simulink subsystem "hardware"  (R2022a)
settings: Solver=VariableStepAuto  StartTime=0.0  StopTime=10.0  RelTol=1e-3
undefined symbols (not defined in the file or in its folder): HS, IO291
libraries: aru_toolbox x5, eeGeneralControl x4, speedgoatlib_IO691 x3, speedgoatlib_IO291 x1
settings Model: Creator=Mechatronics  LastModifiedBy=Mechatronics

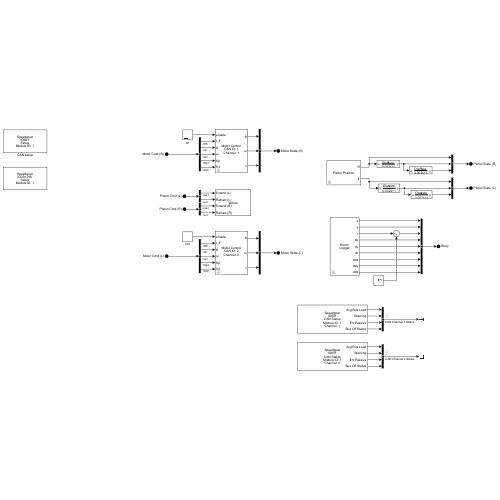
[thumbnail: Simulink's stored preview of the top-level diagram]
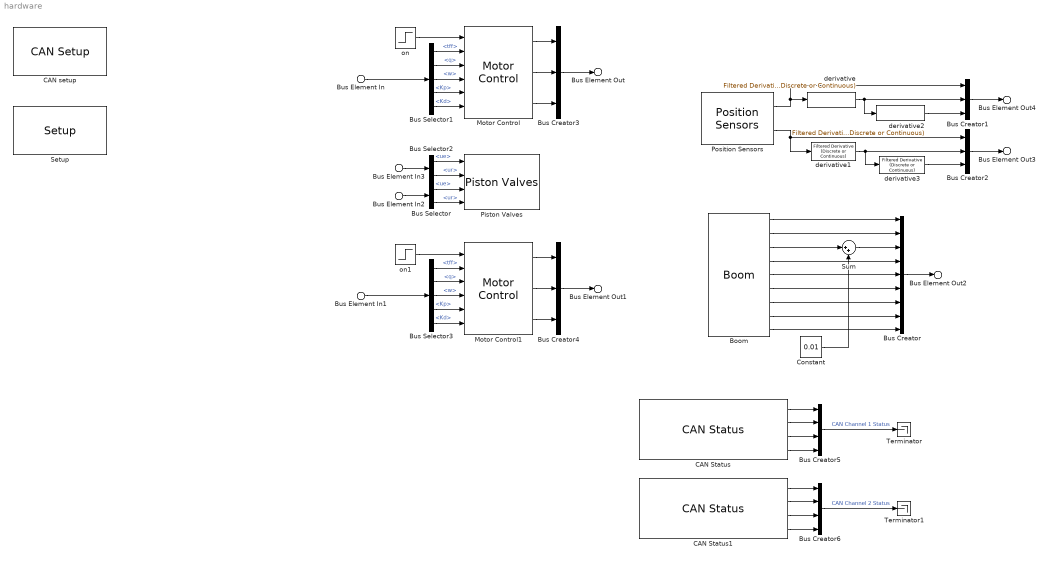
== system hardware ==
  Bus Element In : Inport  PortName=Motor Cmd (R)
  Bus Element In2 : Inport  Port=2  PortName=Piston Cmd (R)
  Bus Element In3 : Inport  Port=3  PortName=Piston Cmd (L)
  Bus Element In1 : Inport  Port=4  PortName=Motor Cmd (L)
  Boom : aru_toolbox/Boom  ts=0.001
      link override Serial Read HW FIFO: pciSlot=-1  board=IO393-50k
      link override Serial Setup: pciSlot=-1  board=IO393-50k
      settings: SourceProductName=ARU Toolbox
  Bus Creator : BusCreator  Inputs=9  OutDataTypeStr=Bus: BodyState  NonVirtualBus=on
      settings: InheritFromInputs=off
  Bus Creator1 : BusCreator  Inputs=3  OutDataTypeStr=Bus: PistonState  NonVirtualBus=on
      settings: InheritFromInputs=off
  Bus Creator2 : BusCreator  Inputs=3  OutDataTypeStr=Bus: PistonState  NonVirtualBus=on
      settings: InheritFromInputs=off
  Bus Creator3 : BusCreator  Inputs=3  OutDataTypeStr=Bus: MotorState  NonVirtualBus=on
      settings: InheritFromInputs=off
  Bus Creator4 : BusCreator  Inputs=3  OutDataTypeStr=Bus: MotorState  NonVirtualBus=on
      settings: InheritFromInputs=off
  Bus Creator5 : BusCreator  Inputs=4  OutDataTypeStr=Bus: CAN  NonVirtualBus=on
      settings: InheritFromInputs=off
  Bus Creator6 : BusCreator  Inputs=4  OutDataTypeStr=Bus: CAN  NonVirtualBus=on
      settings: InheritFromInputs=off
  Bus Selector : BusSelector  OutputSignals=ue,ur
  Bus Selector1 : BusSelector  OutputSignals=tff,q,w,Kp,Kd
  Bus Selector2 : BusSelector  OutputSignals=ue,ur
  Bus Selector3 : BusSelector  OutputSignals=tff,q,w,Kp,Kd
  CAN Status : speedgoatlib_IO691/Legacy/CAN Status  moduleId=1  sampleTime=0.001  channel=1  busRecovery=Auto  arrayOutput=off  controllerCpuLoad=off  controllerLiveCount=off  initModeAct=off  avgBusLoad=on  receiving=off  RxQueueEmpty=off  dataOverrunRcv=off  rxBufferLevel=off  txPending=off  dataOverrunTx=off  txBufferLevel=off  errWarnLimit=on  errPassLimit=on  errBusOff=on  busRecoveryCounter=off  busCouplingErr=off  transceiverErr=off  opMode=off  brp=off  timeSegment1=off  timeSegment2=off  synchronisationJumpWidth=off  dataTSEG1=off  dataTSEG2=off  dataSJW=off  moduleType=691  qtyStatBlk=1  ptIdx=0  isFDMod=0
      settings: SourceProductName=Simulink Real-Time: Speedgoat I/O Blockset
  CAN Status1 : speedgoatlib_IO691/Legacy/CAN Status  moduleId=1  sampleTime=0.001  channel=2  busRecovery=Auto  arrayOutput=off  controllerCpuLoad=off  controllerLiveCount=off  initModeAct=off  avgBusLoad=on  receiving=off  RxQueueEmpty=off  dataOverrunRcv=off  rxBufferLevel=off  txPending=off  dataOverrunTx=off  txBufferLevel=off  errWarnLimit=on  errPassLimit=on  errBusOff=on  busRecoveryCounter=off  busCouplingErr=off  transceiverErr=off  opMode=off  brp=off  timeSegment1=off  timeSegment2=off  synchronisationJumpWidth=off  dataTSEG1=off  dataTSEG2=off  dataSJW=off  moduleType=691  qtyStatBlk=1  ptIdx=0  isFDMod=0
      settings: SourceProductName=Simulink Real-Time: Speedgoat I/O Blockset
  CAN setup : speedgoatlib_IO691/Legacy/CAN Setup   moduletype=IO691  id=1  pciSlot=-1  chn1=CAN (HS)  chn2=CAN (HS)  chn3=Disabled  chn4=Disabled  initStruct=[]  termStruct=[struct('Channel',1,'Protocol','CAN','BRS',0,'Type','Standard','Identifier',1,'Data',[255, 255, 255, 255, 255, 255, 255, 253],'Pause',0.001), struct('Channel',2,'Protocol','CAN','BRS',0,'Type','Standard','Identifier',2,'Data',[255, 255, 255, 255, 255, 255, 255, 253],'Pause',0.001)]  ArbitrationbdrChn1=1.0 MBaud  ArbitrationManbdrChn1=[2,8,31,8]  FdbdrChn1=1.0 MBaud  FdManbdrChn1=[2,8,31,8]  ArbitrationbdrChn2=1.0 MBaud  ArbitrationManbdrChn2=[2,8,31,8]  FdbdrChn2=1.0 MBaud  FdManbdrChn2=[2,8,31,8]  ArbitrationbdrChn3=1.0 MBaud  ArbitrationManbdrChn3=[2,8,31,8]  FdbdrChn3=5.0 MBaud  FdManbdrChn3=[2,2,5,2]  ArbitrationbdrChn4=1.0 MBaud  ArbitrationManbdrChn4=[2,8,31,8]  FdbdrChn4=5.0 MBaud  FdManbdrChn4=[2,2,5,2]  moduleInitValues=[691 1 -1 -1]
      settings: SourceProductName=Simulink Real-Time: Speedgoat I/O Blockset
  Constant : Constant  Value=0.01
  Motor Control : aru_toolbox/Motor Control  id=1  channel=1  offset=0.8294-pi
      settings: SourceProductName=ARU Toolbox
  Motor Control1 : aru_toolbox/Motor Control  id=2  channel=2  offset=-0.5243
      settings: SourceProductName=ARU Toolbox
  Piston Valves : aru_toolbox/Piston Valves  SystemSampleTime=-1  VariantActivationTime=update diagram  Latency=0  AutoFrameSizeCalculation=off
      settings: SourceProductName=ARU Toolbox
  Position Sensors : aru_toolbox/Position Sensors  stroke1=0.07  stroke2=0.07
      settings: SourceProductName=ARU Toolbox
  "Setup " : speedgoatlib_IO291/Setup   parInternalModuleId=1  parPciSlot=-1  parModuleId=1  parModuleType=IO291-HS  parTtlDoChannels=[]  parTtlDoInitValues=1  parTtlDoReset=1  parTtlDiChannels=[1 2 3 4 5]  parIsolDiChannels=[]  parFetDoChannels=[1 2 3 4]  parFetDoInitValues=0  parFetDoReset=1
      settings: SourceProductName=Simulink Real-Time: Speedgoat I/O Blockset
  Sum : Sum  Inputs=|++
  Terminator : Terminator
  Terminator1 : Terminator
  derivative{,1..3} (4 alike) : eeGeneralControl/Filtered Derivative (Discrete or Continuous)  K=1  T=0.002  B=inf  A=-inf  minRatio=2  init_option=Inherited from block input  x0=0  Ts=0.001
      settings: SourceProductBaseCode=PS
  on : Step  SampleTime=0
  on1 : Step  Time=2  SampleTime=0
  Bus Element Out : Outport  PortName=Motor State (R)
  Bus Element Out4 : Outport  Port=2  PortName=Piston State (R)
  Bus Element Out2 : Outport  Port=3  PortName=Body
  Bus Element Out1 : Outport  Port=4  PortName=Motor State (L)
  Bus Element Out3 : Outport  Port=5  PortName=Piston State (L)
  wires:
  Motor Control/2 -> Bus Creator3/2
  Motor Control1/2 -> Bus Creator4/2
  Bus Selector1/1 -> Motor Control/2  "<tff>"
  Bus Creator5/1 -> Terminator/1  "CAN Channel 1 Status"
  derivative2/1 -> Bus Creator1/3
  Bus Selector/1 -> Piston Valves/3  "<ue>"
  Bus Element In/1 -> Bus Selector1/1
  Bus Selector1/4 -> Motor Control/5  "<Kp>"
  Bus Selector/2 -> Piston Valves/4  "<ur>"
  Bus Selector3/4 -> Motor Control1/5  "<Kp>"
  Bus Selector3/2 -> Motor Control1/3  "<q>"
  Bus Selector2/2 -> Piston Valves/2  "<ur>"
  Bus Creator6/1 -> Terminator1/1  "CAN Channel 2 Status"
  CAN Status1/3 -> Bus Creator6/3
  on1/1 -> Motor Control1/1
  Bus Selector2/1 -> Piston Valves/1  "<ue>"
  Bus Element In3/1 -> Bus Selector2/1
  Bus Selector1/3 -> Motor Control/4  "<w>"
  CAN Status1/4 -> Bus Creator6/4
  Bus Selector3/1 -> Motor Control1/2  "<tff>"
  Boom/1 -> Bus Creator/1
  Boom/3 -> Sum/1
  Bus Element In2/1 -> Bus Selector/1
  CAN Status/3 -> Bus Creator5/3
  Bus Creator1/1 -> Bus Element Out4/1
  Boom/7 -> Bus Creator/7
  Boom/5 -> Bus Creator/5
  Boom/6 -> Bus Creator/6
  Bus Creator/1 -> Bus Element Out2/1
  Bus Selector3/5 -> Motor Control1/6  "<Kd>"
  Boom/8 -> Bus Creator/8
  Boom/4 -> Bus Creator/4
  Bus Selector1/2 -> Motor Control/3  "<q>"
  derivative/1 -> derivative2/1, Bus Creator1/2
  derivative3/1 -> Bus Creator2/3
  Bus Creator3/1 -> Bus Element Out/1
  CAN Status/4 -> Bus Creator5/4
  Bus Selector3/3 -> Motor Control1/4  "<w>"
  derivative1/1 -> derivative3/1, Bus Creator2/2
  Boom/2 -> Bus Creator/2
  CAN Status1/2 -> Bus Creator6/2
  Motor Control1/1 -> Bus Creator4/1
  Position Sensors/2 -> derivative1/1, Bus Creator2/1
  Bus Element In1/1 -> Bus Selector3/1
  Motor Control/1 -> Bus Creator3/1
  Bus Selector1/5 -> Motor Control/6  "<Kd>"
  Constant/1 -> Sum/2
  CAN Status/1 -> Bus Creator5/1
  Boom/9 -> Bus Creator/9
  Position Sensors/1 -> Bus Creator1/1, derivative/1
  Motor Control1/3 -> Bus Creator4/3
  Bus Creator4/1 -> Bus Element Out1/1
  Sum/1 -> Bus Creator/3
  on/1 -> Motor Control/1
  CAN Status1/1 -> Bus Creator6/1
  Bus Creator2/1 -> Bus Element Out3/1
  CAN Status/2 -> Bus Creator5/2
  Motor Control/3 -> Bus Creator3/3
